simulink model "sfcndemo_sfun_multiport"  (Simulink 6.0)
settings: Solver=FixedStepDiscrete  StartTime=0.0  StopTime=10.0  RelTol=1e-3
settings Model: Creator=The MathWorks Inc.  LastModifiedBy=batserve  ExtModeTrigMode=oneshot  ExtModeArmWhenConnect=off  ExtModeAutoUpdateStatusClock=off
settings DataIOCC: LimitDataPoints=off
settings OptimizationCC: BooleanDataType=off
settings DebuggingCC: CheckExecutionContextPreStartOutputMsg=on  CheckExecutionContextRuntimeOutputMsg=on  SolverPrmCheckMsg=none
settings HardwareCC: TargetUnknown=on

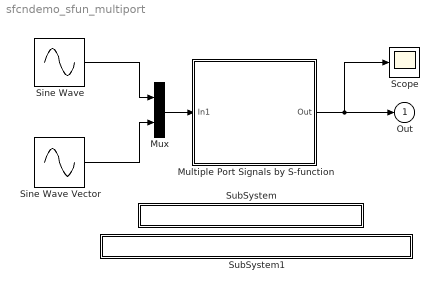
== system sfcndemo_sfun_multiport ==
  Multiple Port Signals by S-function : Subsystem  PropExecContextAcrossSSBoundary=on
      mask Display:
      | disp('S-Function');
      | plot([0 NaN 1 2 3 4 NaN 6 7 8 9 NaN 10 NaN 1 2 3 4 NaN 6 7 8 9 NaN 1 2],[0 NaN 1 1 1 2 NaN 3 3.5 3.5 3.5 NaN 5 NaN 4 4 4 3 NaN 2 1.5 1.5 1.5 NaN 2.5 2.5])
  Mux : Mux  Inputs=2
  Scope : Scope
      settings: TickLabels=on  TimeRange=10  YMin=-15  YMax=15  DataFormat=Array
  Sine Wave : Sin  SampleTime=1
  Sine Wave Vector : Sin  Amplitude=1:3  SampleTime=1
  SubSystem : Subsystem  PropExecContextAcrossSSBoundary=on
      settings: OpenFcn=edit(fullfile(matlabroot,'simulink','src','sfun_multiport.c'))
      mask Display: disp('matlabroot\simulink\src\sfun_multiport.c');
  SubSystem1 : Subsystem  PropExecContextAcrossSSBoundary=on
      settings: OpenFcn=edit(fullfile(matlabroot,'toolbox','simulink','blocks','tlc_c','sfun_multiport.tlc'))
      mask Display: disp('matlabroot\toolbox\simulink\blocks\tlc_c\sfun_multiport.tlc');
  Out : Outport  InitialOutput=0
  wires:
  Sine Wave/1 -> Mux/1
  Sine Wave Vector/1 -> Mux/2
  Mux/1 -> Multiple Port Signals by S-function/1(In1)
  Multiple Port Signals by S-function/1(Out) -> Out/1, Scope/1

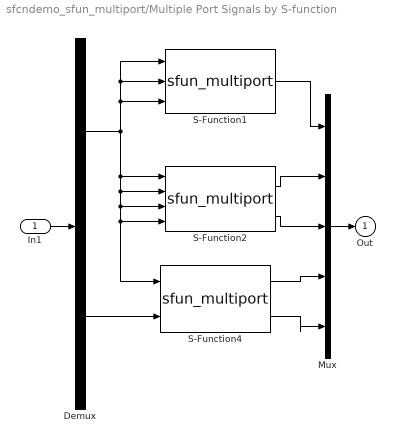
== system sfcndemo_sfun_multiport/Multiple Port Signals by S-function ==
  In1 : Inport  Port=1  PortDimensions=4  LatchInput=off
  Demux : Demux  Outputs=[1 3]
  Mux : Mux  Inputs=5
  S-Function1 : S-Function  FunctionName=sfun_multiport  Parameters=signs,gain,output  mask(S-function: sfun_multiport){signs=+++, gain=4, output=SumTimesGain}
      mask prompts: signs "Input port sign"; output "Output type"
      settings: AttributesFormatString=SumTimesGain
      mask StyleString: edit,edit,popup(SumTimesGain|SumTimesGainAndAverage)
  S-Function2 : S-Function  FunctionName=sfun_multiport  Parameters=signs,gain,output  mask(S-function: sfun_multiport){signs=++++, gain=2, output=SumTimesGainAndAverage}
      mask prompts: signs "Input port sign"; output "Output type"
      settings: AttributesFormatString=SumTimesGainAndAverage
      mask StyleString: edit,edit,popup(SumTimesGain|SumTimesGainAndAverage)
  S-Function4 : S-Function  FunctionName=sfun_multiport  Parameters=signs,gain,output  mask(S-function: sfun_multiport){signs=++, gain=3, output=SumTimesGainAndAverage}
      mask prompts: signs "Input port sign"; output "Output type"
      settings: AttributesFormatString=SumTimesGainAndAverage(Vector)
      mask StyleString: edit,edit,popup(SumTimesGain|SumTimesGainAndAverage)
  Out : Outport  InitialOutput=0
  wires:
  S-Function1/1 -> Mux/1
  S-Function2/2 -> Mux/3
  S-Function4/2 -> Mux/5
  In1/1 -> Demux/1
  Demux/2 -> S-Function4/2
  Demux/1 -> S-Function1/1, S-Function1/2, S-Function1/3, S-Function2/1, S-Function2/3, S-Function4/1, S-Function2/4, S-Function2/2
  S-Function2/1 -> Mux/2
  S-Function4/1 -> Mux/4
  Mux/1 -> Out/1

== system sfcndemo_sfun_multiport/SubSystem ==

== system sfcndemo_sfun_multiport/SubSystem1 ==
